simulink model "untitled1"  (R2023b)
settings: Solver=VariableStepAuto  StartTime=0.0  StopTime=100  RelTol=1e-3
values from neighbouring files (symbols this model uses):
  B1 = 0.001    [untitled.m]
  B2 = 0.001    [untitled.m]
  B_azimut = 0.001 * 8.69    (= 0.00869)    [untitled.m]
  B_elevatie = 0.001 * 1.8    (= 0.0018)    [untitled.m]
  Bp1 = 1    [untitled.m]
  Bp2 = 1    [untitled.m]
  C1 = 0.001    [untitled.m]
  C2 = 0.001    [untitled.m]
  C_azimut = 0    [untitled.m]
  C_elevatie = 0    [untitled.m]
  Dp1 = 1    [untitled.m]
  Dp2 = 1    [untitled.m]
  g = 10    [untitled.m]
  I1 = 1.25    [untitled.m]
  I2 = 2    [untitled.m]
  I_azimut = 0.00414    [untitled.m]
  I_elevatie = 0.00437    [untitled.m]
  K2 = 0.21    [untitled.m]
  Kb2 = 1    [untitled.m]
  Ki2 = 1000    [untitled.m]
  Kw1 = 1    [untitled.m]
  Kw2 = 1    [untitled.m]
  l = 0.33    [untitled.m]
  m = 0.0117    [untitled.m]
  R2 = 1000    [untitled.m]
  u2 = 0.1:0.1:1.2    [untitled.m]
settings Model: Creator=Iustin  LastModifiedBy=Iustin
settings DebuggingCC: UnderSpecifiedDimensionMsg=warning

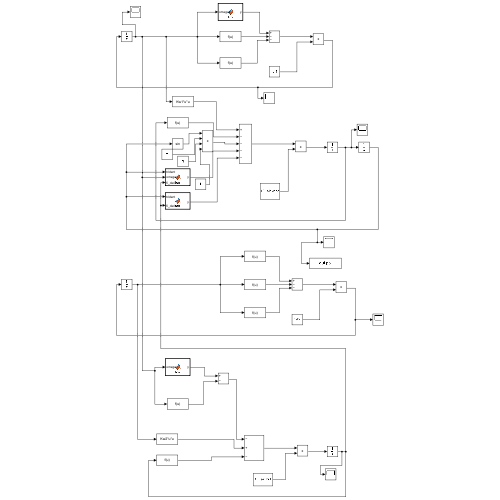
[thumbnail: Simulink's stored preview of the top-level diagram]
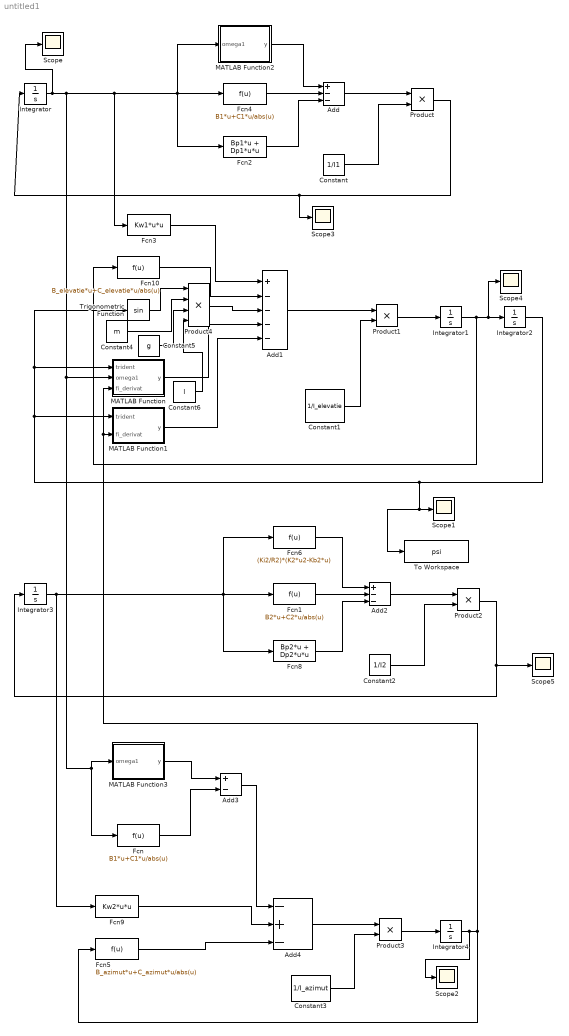
== system untitled1 ==
  Add : Sum  Inputs=+--
  Add1 : Sum  Inputs=+----
  Add2 : Sum  Inputs=+--
  Add3 : Sum  Inputs=+-
  Add4 : Sum  Inputs=-+-
  Constant : Constant  Value=1/I1
  Constant1 : Constant  Value=1/I_elevatie
  Constant2 : Constant  Value=1/I2
  Constant3 : Constant  Value=1/I_azimut
  Constant4 : Constant  Value=m
  Constant5 : Constant  Value=g
  Constant6 : Constant  Value=l
  Fcn : Fcn  Expr=B1*u+C1*u/abs(u)
  Fcn1 : Fcn  Expr=B2*u+C2*u/abs(u)
  Fcn10 : Fcn  Expr=B_elevatie*u+C_elevatie*u/abs(u)
  Fcn2 : Fcn  Expr=Bp1*u + Dp1*u*u
  Fcn3 : Fcn  Expr=Kw1*u*u
  Fcn4 : Fcn  Expr=B1*u+C1*u/abs(u)
  Fcn5 : Fcn  Expr=B_azimut*u+C_azimut*u/abs(u)
  Fcn6 : Fcn  Expr=(Ki2/R2)*(K2*u2-Kb2*u)
  Fcn8 : Fcn  Expr=Bp2*u + Dp2*u*u
  Fcn9 : Fcn  Expr=Kw2*u*u
  Integrator{,1..4} (5 alike) : Integrator  InitialCondition=1
  MATLAB Function : MATLAB Function  TreatAsAtomicUnit=on
  MATLAB Function1 : MATLAB Function  TreatAsAtomicUnit=on
  MATLAB Function2 : MATLAB Function  TreatAsAtomicUnit=on
  MATLAB Function3 : MATLAB Function  TreatAsAtomicUnit=on
  Product{,1..3} (4 alike) : Product
  Product4 : Product  Inputs=4
  Scope{,1..5} (6 alike) : Scope
  To Workspace : ToWorkspace  VariableName=psi  SampleTime=-1
  Trigonometric Function : Trigonometry
  wires:
  Add/1 -> Product/1
  Constant/1 -> Product/2
  Integrator/1 -> Scope/1, Fcn3/1, Fcn4/1, Fcn2/1, MATLAB Function2/1(omega1), MATLAB Function/2(omega1), Fcn/1, MATLAB Function3/1(omega1)
  Product/1 -> Scope3/1, Integrator/1
  Fcn3/1 -> Add1/1
  MATLAB Function/1(y) -> Add1/4
  MATLAB Function1/1(y) -> Add1/5
  Add1/1 -> Product1/1
  Constant1/1 -> Product1/2
  Product1/1 -> Integrator1/1
  Integrator1/1 -> Fcn10/1, Scope4/1, Integrator2/1
  Integrator2/1 -> To Workspace/1, Scope1/1, Trigonometric Function/1, MATLAB Function/1(trident), MATLAB Function1/1(trident)
  Constant2/1 -> Product2/2
  Add2/1 -> Product2/1
  Fcn6/1 -> Add2/1
  Product2/1 -> Scope5/1, Integrator3/1
  Fcn8/1 -> Add2/3
  Integrator3/1 -> Fcn9/1, Fcn1/1, Fcn8/1, Fcn6/1
  MATLAB Function2/1(y) -> Add/1
  MATLAB Function3/1(y) -> Add3/1
  Fcn9/1 -> Add4/2
  Add3/1 -> Add4/1
  Add4/1 -> Product3/1
  Constant3/1 -> Product3/2
  Product3/1 -> Integrator4/1
  Integrator4/1 -> Fcn5/1, MATLAB Function/3(fi_derivat), MATLAB Function1/2(fi_derivat), Scope2/1
  Fcn/1 -> Add3/2
  Fcn1/1 -> Add2/2
  Fcn2/1 -> Add/3
  Fcn4/1 -> Add/2
  Fcn5/1 -> Add4/3
  Fcn10/1 -> Add1/2
  Product4/1 -> Add1/3
  Trigonometric Function/1 -> Product4/1
  Constant4/1 -> Product4/2
  Constant5/1 -> Product4/3
  Constant6/1 -> Product4/4

== matlab function untitled1/MATLAB Function ==
  data: trident input; y output; omega1 input; fi_derivat input
function y = fcn(trident,omega1,fi_derivat)
%codegen


K_gyro = 0.015



y = K_gyro * cos(trident) * omega1 * omega1 * fi_derivat;

== matlab function untitled1/MATLAB Function2 ==
  data: y output; omega1 input

function y = fcn( omega1)
%codegen


K1 = 0.53;
R1 = 1000;
Ki1 = 1000;
Kb1 = 1;
u1=0.1


y = (Ki1 / R1) * (K1 * u1 - Kb1 * omega1);

== matlab function untitled1/MATLAB Function3 ==
  data: y output; omega1 input
function y = fcn( omega1)


K1 = 0.53
R1 = 1000
Ki1 = 1000
Kb1 = 1
u1=0.1


y = (Ki1/R1)*(K1 * u1 - Kb1 * omega1);

== matlab function untitled1/MATLAB Function1 ==
  data: trident input; y output; fi_derivat input
function y = fcn(trident, fi_derivat)
%codegen


m = 0.0117
l = 0.33
g = 10


y = (m*l/2) * sin(2*trident) * fi_derivat * fi_derivat;
